simulink model "Motorcontrol_P"  (R2025b)
settings: Solver=VariableStepAuto  StartTime=0.0  StopTime=0.2  RelTol=1e-3
undefined symbols (not defined in the file): cm, D, J, Kp, L, R
settings Model: Creator=yashd  LastModifiedBy=yashd

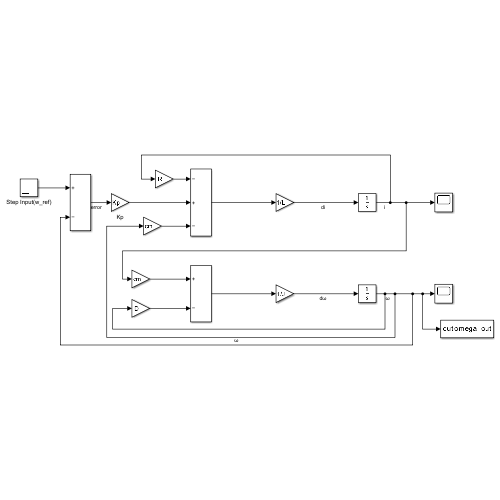
[thumbnail: Simulink's stored preview of the top-level diagram]
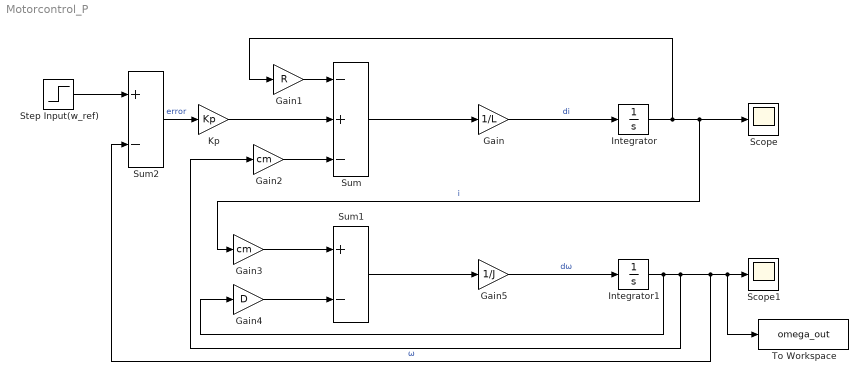
== system Motorcontrol_P ==
  Gain : Gain  Gain=1/L
  Gain1 : Gain  Gain=R
  Gain2 : Gain  Gain=cm
  Gain3 : Gain  Gain=cm
  Gain4 : Gain  Gain=D
  Gain5 : Gain  Gain=1/J
  Integrator : Integrator
  Integrator1 : Integrator
  Kp : Gain  Gain=Kp
  Scope : Scope
      settings: ActiveDisplayYMinimum=-0.51588134059042334  ActiveDisplayYMaximum=1.7924602428520262  DataLoggingVariableName=xx
  Scope1 : Scope
      settings: ActiveDisplayYMinimum=145.95262108913147  ActiveDisplayYMaximum=229.39997004066765  DataLoggingVariableName=xy
  Step Input(w_ref) : Step  Time=0  Before=1  After=200  SampleTime=0
  Sum : Sum  Inputs=-+-
  Sum1 : Sum  Inputs=+-
  Sum2 : Sum  Inputs=+-
  To Workspace : ToWorkspace  VariableName=omega_out  SaveFormat=Structure With Time  SampleTime=-1
  wires:
  Sum/1 -> Gain/1
  Gain/1 -> Integrator/1  "di"
  Integrator/1 -> Gain3/1, Scope/1, Gain1/1  "i"
  Gain5/1 -> Integrator1/1  "dω"
  Sum1/1 -> Gain5/1
  Integrator1/1 -> Sum2/2, To Workspace/1, Scope1/1, Gain2/1, Gain4/1  "ω"
  Gain3/1 -> Sum1/1
  Gain4/1 -> Sum1/2
  Step Input(w_ref)/1 -> Sum2/1
  Sum2/1 -> Kp/1  "error"
  Gain2/1 -> Sum/3
  Gain1/1 -> Sum/1
  Kp/1 -> Sum/2
